simulink model "conv5x5_video_ex"  (Simulink 7.7)
settings: Solver=VariableStepDiscrete  SolverMode=SingleTasking  StartTime=0.0  StopTime=1000  RelTol=1e-3
undefined symbols (not defined in the file or in its folder): xrbsImage_r3
libraries: xbsIndex_r4 x204, xrbsImage_r4 x1, xbsCopyrightNotice_r4 x1
(part 3 of 3)

== system conv5x5_video_ex/5x5_filter/5x5Filter/n-tap MAC FIR Filter2/MAC Engine ==
  note: The Multiplier block is implemented using Virtex-II  dedicated multipliers.
      | Enabling the 'Pipeline to Greatest Extent Possible' mask configuration
      | parameter ensures the internal pipeline stages of the dedicated
      | multipliers are used.
  note: This subsystem implements a multiply-accumulate engine.
  note: Upon reset, the accumulator reinitializes to its current input value
      | rather than zero, which allows the MAC engine to stream data without
      | stalling for one sample period.
  note: The precision required for the multiplier and the accumulator is a
      | function of the filter taps (coefficients) and the number of taps. Since
      | these are fixed at design time, it is possible to tailor the hardware resources
      | to the filter specification.  The multiplier need only have enough  bits to
      | compute the product of the largest magnitude coefficient and the largest
      | magnitude data input value.   That is,
      |
      |         mult_nbits = ceil(log2(max(abs(coef*2^coef_binpt))))+input_nbits + 1;
      |         mult_binpt = input_binpt+coef_binpt;
      |
      | Similarly, the accumulator need only have sufficient precision to accumulate
      | maximal input against the filter taps.
      |
      |         acc_nbits = ceil(log2(sum(abs(coef*2^coef_binpt)))) + input_nbits + 1;
      |         acc_binpt = mult_binpt;
      |
      | These variables are passed to the blocks as mask parameters.
  a : Inport
  b : Inport  Port=2
  rst : Inport  Port=3
  Accumulator : xbsIndex_r4/Accumulator  operation=Add  n_bits=ceil(log2(max(1,sum(abs(coef*2^coef_bin_pt)))))+smpl_n_bits + 1  overflow=Wrap  scale=1  rst=on  hasbypass=on  en=off  dbl_ovrd=off  use_behavioral_HDL=on  implementation=Fabric  block_type=accum
      settings: infoedit="Adder or subtractor-based accumulator.   Output type and binary point position match the input.<P><P>Hardware notes: When \"Reinitialize with Input 'b' on Reset\" is selected, the accumulator is forced to run at the system rate even if the input 'b' is running at a slower rate."  xl_area=[0, 0, 0, 0, 0, 0, 0]  block_version=VER_STRING_GOES_HERE
  Mult : xbsIndex_r4/Mult  precision=User Defined  arith_type="Signed  (2's comp)"  n_bits=max(ceil(log2(max(1,max(abs(coef*2^coef_bin_pt)))))+smpl_n_bits + 1,smpl_bin_pt+coef_bin_pt)  bin_pt=smpl_bin_pt+coef_bin_pt  quantization=Truncate  overflow=Wrap  en=off  latency=2  dbl_ovrd=off  use_behavioral_HDL=off  opt=Speed  use_embedded=on  optimum_pipeline=off  pipeline=on  use_rpm=on  placement_style=Rectangular shape  block_type=mult
      settings: infoedit=Multiplies two values.<P><P>Hardware notes: To use the internal pipeline stage of the dedicated multiplier you must select 'Pipeline to Greatest Extent Possible'.  xl_area=[0, 0, 0, 0, 0, 0, 0]  block_version=VER_STRING_GOES_HERE
  q : Outport
  wires:
  rst/1 -> Accumulator/2
  b/1 -> Mult/2
  Accumulator/1 -> q/1
  a/1 -> Mult/1
  Mult/1 -> Accumulator/1

== system conv5x5_video_ex/5x5_filter/5x5Filter/n-tap MAC FIR Filter3/Coefficient RAM ==
  coef_in : Inport
  load : Inport  Port=2
  addr : Inport  Port=3
  Concat : xbsIndex_r4/Concat  num_inputs=2  dbl_ovrd=off  block_type=concat
      settings: block_version=VER_STRING_GOES_HERE
  Concat1 : xbsIndex_r4/Concat  num_inputs=2  dbl_ovrd=off  block_type=concat
      settings: block_version=VER_STRING_GOES_HERE
  Constant : xbsIndex_r4/Constant  const=length(coef)-1  gui_display_data_type=Fixed-point  arith_type=Unsigned  n_bits=ceil(log2(length(coef)))  bin_pt=0  preci_type=Single  exp_width=8  frac_width=24  explicit_period=off  period=1  equ=P=C  opselect=C  inp2=PCIN>>17  opr=+  inp1=P  carry=CIN  dbl_ovrd=off  block_type=constant
      settings: block_version=VER_STRING_GOES_HERE
  Convert : xbsIndex_r4/Convert  gui_display_data_type=Fixed-point  arith_type="Signed  (2's comp)"  n_bits=coef_n_bits  bin_pt=coef_bin_pt  float_type=Single  exp_bits=8  fraction_bits=24  quantization=Truncate  overflow=Wrap  en=off  latency=0  dbl_ovrd=off  pipeline=off  block_type=convert
      settings: infoedit=The input is presented at the output after quantization and overflow effects.<P><P>Hardware notes: Additional hardware is used when rounding or saturation is selected and output width is less than the input width.  xl_area=[0, 0, 0, 0, 0, 0, 0]  block_version=VER_STRING_GOES_HERE
  Counter1 : xbsIndex_r4/Counter  cnt_type=Count Limited  cnt_to=length(coef)-1  operation=Up  start_count=0  cnt_by_val=1  arith_type=Unsigned  n_bits=ceil(log2(length(coef)))  bin_pt=0  load_pin=off  rst=off  en=on  explicit_period=on  period=smpl_period/length(coef)  dbl_ovrd=off  use_behavioral_HDL=off  implementation=Fabric  use_rpm=off  block_type=counter
      settings: infoedit="Configurable up, down and up/down counter.<P><P>Hardware notes: Free running counters are the least expensive in hardware.  A count limited counter is implemented by combining a counter with a comparator."  xl_area=[0, 0, 0, 0, 0, 0, 0]  block_version=VER_STRING_GOES_HERE
  Dual Port RAM : xbsIndex_r4/Dual Port RAM  depth=(2^ceil(log2(length(coef))))*2  initVector=coef  distributed_mem=Distributed memory  init_a=0  init_b=0  rst_a=off  rst_b=off  en_a=off  en_b=off  latency=1  write_mode_A=Read After Write  write_mode_B=Read After Write  dbl_ovrd=off  optimize=Area  use_rpm=off  block_type=dpram
      settings: xl_area=[0, 0, 0, 0, 0, 0, 0]  block_version=VER_STRING_GOES_HERE
  Inverter : xbsIndex_r4/Inverter  en=off  latency=0  dbl_ovrd=off  block_type=inv
      settings: xl_area=[0, 0, 0, 0, 0, 0, 0]  block_version=VER_STRING_GOES_HERE
  Relational : xbsIndex_r4/Relational  mode=a=b  en=off  latency=0  dbl_ovrd=off  block_type=relational
      settings: xl_area=[0, 0, 0, 0, 0, 0, 0]  block_version=VER_STRING_GOES_HERE
  T Flip Flop : Subsystem
  Terminator : Terminator
  coef_out : Outport
  wires:
  Inverter/1 -> Concat/1
  T Flip Flop/1(q) -> Concat1/1, Inverter/1
  Relational/1 -> T Flip Flop/1(t)
  Constant/1 -> Relational/2
  Concat1/1 -> Dual Port RAM/4
  addr/1 -> Concat1/2
  Concat/1 -> Dual Port RAM/1
  Convert/1 -> Dual Port RAM/2
  Dual Port RAM/1 -> Terminator/1
  Counter1/1 -> Relational/1, Concat/2
  load/1 -> Dual Port RAM/3, Counter1/1
  coef_in/1 -> Convert/1
  Dual Port RAM/2 -> coef_out/1

== system conv5x5_video_ex/5x5_filter/5x5Filter/n-tap MAC FIR Filter3/MAC Engine ==
  note: The precision required for the multiplier and the accumulator is a
      | function of the filter taps (coefficients) and the number of taps. Since
      | these are fixed at design time, it is possible to tailor the hardware resources
      | to the filter specification.  The multiplier need only have enough  bits to
      | compute the product of the largest magnitude coefficient and the largest
      | magnitude data input value.   That is,
      |
      |         mult_nbits = ceil(log2(max(abs(coef*2^coef_binpt))))+input_nbits + 1;
      |         mult_binpt = input_binpt+coef_binpt;
      |
      | Similarly, the accumulator need only have sufficient precision to accumulate
      | maximal input against the filter taps.
      |
      |         acc_nbits = ceil(log2(sum(abs(coef*2^coef_binpt)))) + input_nbits + 1;
      |         acc_binpt = mult_binpt;
      |
      | These variables are passed to the blocks as mask parameters.
  note: Upon reset, the accumulator reinitializes to its current input value
      | rather than zero, which allows the MAC engine to stream data without
      | stalling for one sample period.
  note: This subsystem implements a multiply-accumulate engine.
  note: The Multiplier block is implemented using Virtex-II  dedicated multipliers.
      | Enabling the 'Pipeline to Greatest Extent Possible' mask configuration
      | parameter ensures the internal pipeline stages of the dedicated
      | multipliers are used.
  a : Inport
  b : Inport  Port=2
  rst : Inport  Port=3
  Accumulator : xbsIndex_r4/Accumulator  operation=Add  n_bits=ceil(log2(max(1,sum(abs(coef*2^coef_bin_pt)))))+smpl_n_bits + 1  overflow=Wrap  scale=1  rst=on  hasbypass=on  en=off  dbl_ovrd=off  use_behavioral_HDL=on  implementation=Fabric  block_type=accum
      settings: infoedit="Adder or subtractor-based accumulator.   Output type and binary point position match the input.<P><P>Hardware notes: When \"Reinitialize with Input 'b' on Reset\" is selected, the accumulator is forced to run at the system rate even if the input 'b' is running at a slower rate."  xl_area=[0, 0, 0, 0, 0, 0, 0]  block_version=VER_STRING_GOES_HERE
  Mult : xbsIndex_r4/Mult  precision=User Defined  arith_type="Signed  (2's comp)"  n_bits=max(ceil(log2(max(1,max(abs(coef*2^coef_bin_pt)))))+smpl_n_bits + 1,smpl_bin_pt+coef_bin_pt)  bin_pt=smpl_bin_pt+coef_bin_pt  quantization=Truncate  overflow=Wrap  en=off  latency=2  dbl_ovrd=off  use_behavioral_HDL=off  opt=Speed  use_embedded=on  optimum_pipeline=off  pipeline=on  use_rpm=on  placement_style=Rectangular shape  block_type=mult
      settings: infoedit=Multiplies two values.<P><P>Hardware notes: To use the internal pipeline stage of the dedicated multiplier you must select 'Pipeline to Greatest Extent Possible'.  xl_area=[0, 0, 0, 0, 0, 0, 0]  block_version=VER_STRING_GOES_HERE
  q : Outport
  wires:
  Mult/1 -> Accumulator/1
  a/1 -> Mult/1
  Accumulator/1 -> q/1
  b/1 -> Mult/2
  rst/1 -> Accumulator/2

== system conv5x5_video_ex/5x5_filter/5x5Filter/n-tap MAC FIR Filter4/Coefficient RAM ==
  coef_in : Inport
  load : Inport  Port=2
  addr : Inport  Port=3
  Concat : xbsIndex_r4/Concat  num_inputs=2  dbl_ovrd=off  block_type=concat
      settings: block_version=VER_STRING_GOES_HERE
  Concat1 : xbsIndex_r4/Concat  num_inputs=2  dbl_ovrd=off  block_type=concat
      settings: block_version=VER_STRING_GOES_HERE
  Constant : xbsIndex_r4/Constant  const=length(coef)-1  gui_display_data_type=Fixed-point  arith_type=Unsigned  n_bits=ceil(log2(length(coef)))  bin_pt=0  preci_type=Single  exp_width=8  frac_width=24  explicit_period=off  period=1  equ=P=C  opselect=C  inp2=PCIN>>17  opr=+  inp1=P  carry=CIN  dbl_ovrd=off  block_type=constant
      settings: block_version=VER_STRING_GOES_HERE
  Convert : xbsIndex_r4/Convert  gui_display_data_type=Fixed-point  arith_type="Signed  (2's comp)"  n_bits=coef_n_bits  bin_pt=coef_bin_pt  float_type=Single  exp_bits=8  fraction_bits=24  quantization=Truncate  overflow=Wrap  en=off  latency=0  dbl_ovrd=off  pipeline=off  block_type=convert
      settings: infoedit=The input is presented at the output after quantization and overflow effects.<P><P>Hardware notes: Additional hardware is used when rounding or saturation is selected and output width is less than the input width.  xl_area=[0, 0, 0, 0, 0, 0, 0]  block_version=VER_STRING_GOES_HERE
  Counter1 : xbsIndex_r4/Counter  cnt_type=Count Limited  cnt_to=length(coef)-1  operation=Up  start_count=0  cnt_by_val=1  arith_type=Unsigned  n_bits=ceil(log2(length(coef)))  bin_pt=0  load_pin=off  rst=off  en=on  explicit_period=on  period=smpl_period/length(coef)  dbl_ovrd=off  use_behavioral_HDL=off  implementation=Fabric  use_rpm=off  block_type=counter
      settings: infoedit="Configurable up, down and up/down counter.<P><P>Hardware notes: Free running counters are the least expensive in hardware.  A count limited counter is implemented by combining a counter with a comparator."  xl_area=[0, 0, 0, 0, 0, 0, 0]  block_version=VER_STRING_GOES_HERE
  Dual Port RAM : xbsIndex_r4/Dual Port RAM  depth=(2^ceil(log2(length(coef))))*2  initVector=coef  distributed_mem=Distributed memory  init_a=0  init_b=0  rst_a=off  rst_b=off  en_a=off  en_b=off  latency=1  write_mode_A=Read After Write  write_mode_B=Read After Write  dbl_ovrd=off  optimize=Area  use_rpm=off  block_type=dpram
      settings: xl_area=[0, 0, 0, 0, 0, 0, 0]  block_version=VER_STRING_GOES_HERE
  Inverter : xbsIndex_r4/Inverter  en=off  latency=0  dbl_ovrd=off  block_type=inv
      settings: xl_area=[0, 0, 0, 0, 0, 0, 0]  block_version=VER_STRING_GOES_HERE
  Relational : xbsIndex_r4/Relational  mode=a=b  en=off  latency=0  dbl_ovrd=off  block_type=relational
      settings: xl_area=[0, 0, 0, 0, 0, 0, 0]  block_version=VER_STRING_GOES_HERE
  T Flip Flop : Subsystem
  Terminator : Terminator
  coef_out : Outport
  wires:
  Dual Port RAM/2 -> coef_out/1
  coef_in/1 -> Convert/1
  load/1 -> Counter1/1, Dual Port RAM/3
  Counter1/1 -> Concat/2, Relational/1
  Dual Port RAM/1 -> Terminator/1
  Convert/1 -> Dual Port RAM/2
  Concat/1 -> Dual Port RAM/1
  addr/1 -> Concat1/2
  Concat1/1 -> Dual Port RAM/4
  Constant/1 -> Relational/2
  Relational/1 -> T Flip Flop/1(t)
  T Flip Flop/1(q) -> Inverter/1, Concat1/1
  Inverter/1 -> Concat/1

== system conv5x5_video_ex/5x5_filter/5x5Filter/n-tap MAC FIR Filter4/MAC Engine ==
  note: The Multiplier block is implemented using Virtex-II  dedicated multipliers.
      | Enabling the 'Pipeline to Greatest Extent Possible' mask configuration
      | parameter ensures the internal pipeline stages of the dedicated
      | multipliers are used.
  note: This subsystem implements a multiply-accumulate engine.
  note: Upon reset, the accumulator reinitializes to its current input value
      | rather than zero, which allows the MAC engine to stream data without
      | stalling for one sample period.
  note: The precision required for the multiplier and the accumulator is a
      | function of the filter taps (coefficients) and the number of taps. Since
      | these are fixed at design time, it is possible to tailor the hardware resources
      | to the filter specification.  The multiplier need only have enough  bits to
      | compute the product of the largest magnitude coefficient and the largest
      | magnitude data input value.   That is,
      |
      |         mult_nbits = ceil(log2(max(abs(coef*2^coef_binpt))))+input_nbits + 1;
      |         mult_binpt = input_binpt+coef_binpt;
      |
      | Similarly, the accumulator need only have sufficient precision to accumulate
      | maximal input against the filter taps.
      |
      |         acc_nbits = ceil(log2(sum(abs(coef*2^coef_binpt)))) + input_nbits + 1;
      |         acc_binpt = mult_binpt;
      |
      | These variables are passed to the blocks as mask parameters.
  a : Inport
  b : Inport  Port=2
  rst : Inport  Port=3
  Accumulator : xbsIndex_r4/Accumulator  operation=Add  n_bits=ceil(log2(max(1,sum(abs(coef*2^coef_bin_pt)))))+smpl_n_bits + 1  overflow=Wrap  scale=1  rst=on  hasbypass=on  en=off  dbl_ovrd=off  use_behavioral_HDL=on  implementation=Fabric  block_type=accum
      settings: infoedit="Adder or subtractor-based accumulator.   Output type and binary point position match the input.<P><P>Hardware notes: When \"Reinitialize with Input 'b' on Reset\" is selected, the accumulator is forced to run at the system rate even if the input 'b' is running at a slower rate."  xl_area=[0, 0, 0, 0, 0, 0, 0]  block_version=VER_STRING_GOES_HERE
  Mult : xbsIndex_r4/Mult  precision=User Defined  arith_type="Signed  (2's comp)"  n_bits=max(ceil(log2(max(1,max(abs(coef*2^coef_bin_pt)))))+smpl_n_bits + 1,smpl_bin_pt+coef_bin_pt)  bin_pt=smpl_bin_pt+coef_bin_pt  quantization=Truncate  overflow=Wrap  en=off  latency=2  dbl_ovrd=off  use_behavioral_HDL=off  opt=Speed  use_embedded=on  optimum_pipeline=off  pipeline=on  use_rpm=on  placement_style=Rectangular shape  block_type=mult
      settings: infoedit=Multiplies two values.<P><P>Hardware notes: To use the internal pipeline stage of the dedicated multiplier you must select 'Pipeline to Greatest Extent Possible'.  xl_area=[0, 0, 0, 0, 0, 0, 0]  block_version=VER_STRING_GOES_HERE
  q : Outport
  wires:
  rst/1 -> Accumulator/2
  b/1 -> Mult/2
  Accumulator/1 -> q/1
  a/1 -> Mult/1
  Mult/1 -> Accumulator/1

== system conv5x5_video_ex/5x5_filter/5x5Filter/n-tap MAC FIR Filter/Coefficient RAM/T Flip Flop ==
  t : Inport
  Convert1 : xbsIndex_r4/Convert  gui_display_data_type=Fixed-point  arith_type=Unsigned  n_bits=1  bin_pt=0  float_type=Single  exp_bits=8  fraction_bits=24  quantization=Truncate  overflow=Wrap  en=off  latency=0  dbl_ovrd=off  pipeline=off  block_type=convert
      settings: infoedit=The input is presented at the output after quantization and overflow effects.<P><P>Hardware notes: Additional hardware is used when rounding or saturation is selected and output width is less than the input width.  xl_area=[0, 0, 0, 0, 0, 0, 0]  block_version=VER_STRING_GOES_HERE
  Inverter : xbsIndex_r4/Inverter  en=off  latency=0  dbl_ovrd=off  block_type=inv
      settings: xl_area=[0, 0, 0, 0, 0, 0, 0]  block_version=VER_STRING_GOES_HERE
  Register : xbsIndex_r4/Register  init=0  rst=off  en=on  dbl_ovrd=off  block_type=register
      settings: xl_area=[0, 0, 0, 0, 0, 0, 0]  block_version=VER_STRING_GOES_HERE
  q : Outport
  wires:
  Register/1 -> q/1, Convert1/1
  Inverter/1 -> Register/1
  Convert1/1 -> Inverter/1
  t/1 -> Register/2

== system conv5x5_video_ex/5x5_filter/5x5Filter/n-tap MAC FIR Filter1/Coefficient RAM/T Flip Flop ==
  t : Inport
  Convert1 : xbsIndex_r4/Convert  gui_display_data_type=Fixed-point  arith_type=Unsigned  n_bits=1  bin_pt=0  float_type=Single  exp_bits=8  fraction_bits=24  quantization=Truncate  overflow=Wrap  en=off  latency=0  dbl_ovrd=off  pipeline=off  block_type=convert
      settings: infoedit=The input is presented at the output after quantization and overflow effects.<P><P>Hardware notes: Additional hardware is used when rounding or saturation is selected and output width is less than the input width.  xl_area=[0, 0, 0, 0, 0, 0, 0]  block_version=VER_STRING_GOES_HERE
  Inverter : xbsIndex_r4/Inverter  en=off  latency=0  dbl_ovrd=off  block_type=inv
      settings: xl_area=[0, 0, 0, 0, 0, 0, 0]  block_version=VER_STRING_GOES_HERE
  Register : xbsIndex_r4/Register  init=0  rst=off  en=on  dbl_ovrd=off  block_type=register
      settings: xl_area=[0, 0, 0, 0, 0, 0, 0]  block_version=VER_STRING_GOES_HERE
  q : Outport
  wires:
  t/1 -> Register/2
  Convert1/1 -> Inverter/1
  Inverter/1 -> Register/1
  Register/1 -> Convert1/1, q/1

== system conv5x5_video_ex/5x5_filter/5x5Filter/n-tap MAC FIR Filter2/Coefficient RAM/T Flip Flop ==
  t : Inport
  Convert1 : xbsIndex_r4/Convert  gui_display_data_type=Fixed-point  arith_type=Unsigned  n_bits=1  bin_pt=0  float_type=Single  exp_bits=8  fraction_bits=24  quantization=Truncate  overflow=Wrap  en=off  latency=0  dbl_ovrd=off  pipeline=off  block_type=convert
      settings: infoedit=The input is presented at the output after quantization and overflow effects.<P><P>Hardware notes: Additional hardware is used when rounding or saturation is selected and output width is less than the input width.  xl_area=[0, 0, 0, 0, 0, 0, 0]  block_version=VER_STRING_GOES_HERE
  Inverter : xbsIndex_r4/Inverter  en=off  latency=0  dbl_ovrd=off  block_type=inv
      settings: xl_area=[0, 0, 0, 0, 0, 0, 0]  block_version=VER_STRING_GOES_HERE
  Register : xbsIndex_r4/Register  init=0  rst=off  en=on  dbl_ovrd=off  block_type=register
      settings: xl_area=[0, 0, 0, 0, 0, 0, 0]  block_version=VER_STRING_GOES_HERE
  q : Outport
  wires:
  Register/1 -> q/1, Convert1/1
  Inverter/1 -> Register/1
  Convert1/1 -> Inverter/1
  t/1 -> Register/2

== system conv5x5_video_ex/5x5_filter/5x5Filter/n-tap MAC FIR Filter3/Coefficient RAM/T Flip Flop ==
  t : Inport
  Convert1 : xbsIndex_r4/Convert  gui_display_data_type=Fixed-point  arith_type=Unsigned  n_bits=1  bin_pt=0  float_type=Single  exp_bits=8  fraction_bits=24  quantization=Truncate  overflow=Wrap  en=off  latency=0  dbl_ovrd=off  pipeline=off  block_type=convert
      settings: infoedit=The input is presented at the output after quantization and overflow effects.<P><P>Hardware notes: Additional hardware is used when rounding or saturation is selected and output width is less than the input width.  xl_area=[0, 0, 0, 0, 0, 0, 0]  block_version=VER_STRING_GOES_HERE
  Inverter : xbsIndex_r4/Inverter  en=off  latency=0  dbl_ovrd=off  block_type=inv
      settings: xl_area=[0, 0, 0, 0, 0, 0, 0]  block_version=VER_STRING_GOES_HERE
  Register : xbsIndex_r4/Register  init=0  rst=off  en=on  dbl_ovrd=off  block_type=register
      settings: xl_area=[0, 0, 0, 0, 0, 0, 0]  block_version=VER_STRING_GOES_HERE
  q : Outport
  wires:
  t/1 -> Register/2
  Convert1/1 -> Inverter/1
  Inverter/1 -> Register/1
  Register/1 -> Convert1/1, q/1

== system conv5x5_video_ex/5x5_filter/5x5Filter/n-tap MAC FIR Filter4/Coefficient RAM/T Flip Flop ==
  t : Inport
  Convert1 : xbsIndex_r4/Convert  gui_display_data_type=Fixed-point  arith_type=Unsigned  n_bits=1  bin_pt=0  float_type=Single  exp_bits=8  fraction_bits=24  quantization=Truncate  overflow=Wrap  en=off  latency=0  dbl_ovrd=off  pipeline=off  block_type=convert
      settings: infoedit=The input is presented at the output after quantization and overflow effects.<P><P>Hardware notes: Additional hardware is used when rounding or saturation is selected and output width is less than the input width.  xl_area=[0, 0, 0, 0, 0, 0, 0]  block_version=VER_STRING_GOES_HERE
  Inverter : xbsIndex_r4/Inverter  en=off  latency=0  dbl_ovrd=off  block_type=inv
      settings: xl_area=[0, 0, 0, 0, 0, 0, 0]  block_version=VER_STRING_GOES_HERE
  Register : xbsIndex_r4/Register  init=0  rst=off  en=on  dbl_ovrd=off  block_type=register
      settings: xl_area=[0, 0, 0, 0, 0, 0, 0]  block_version=VER_STRING_GOES_HERE
  q : Outport
  wires:
  Register/1 -> q/1, Convert1/1
  Inverter/1 -> Register/1
  Convert1/1 -> Inverter/1
  t/1 -> Register/2
